simulink model "system_input_18a"  (R2018a)
settings: Solver=FixedStepAuto  StartTime=0.0  StopTime=95  FixedStep=0.05  RelTol=1e-3
libraries: simulink x1
settings Model: Creator=zeiph  LastModifiedBy=zeiph
settings DataIOCC: ReturnWorkspaceOutputs=on
settings SFSimCC: SimUseLocalCustomCode=on
settings RTWCC: RTWUseLocalCustomCode=on

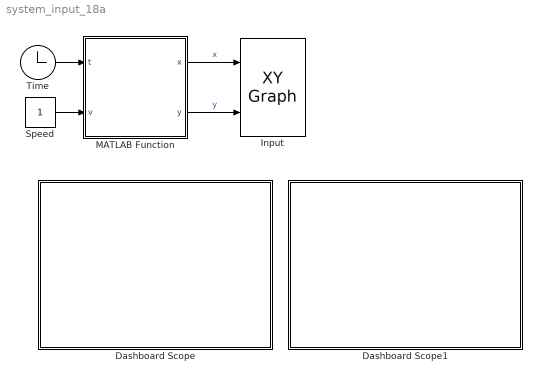
== system system_input_18a ==
  Dashboard Scope : Subsystem  DialogController=hmiCreateDDGDialog  IsWebBlock=on  mask(MWDashboardBlock){webBlockId=c4dcd67c-61d0-45f4-9390-1c8481d4d7a9, webBlockType=sdiscope, ShowInLibBrowser=on, ShowInitialText=on, HMISrcModelName=system_input_18a}
      mask prompts: webBlockId "WebBlock Id"; webBlockType "WebBlock Type"; HMISrcModelName "Source Model"
      mask help: Traces signals on the dashboard scope during simulation.
      mask Help: helpview([docroot '/mapfiles/simulink.map'], 'hmi_scope')
      mask Display:
      | if strcmp(get_param(bdroot(gcb),'BlockDiagramType'),'library')
      |  image([(matlabroot) '/toolbox/simulink/hmi/icons/SDIScope.png'])
      | end
  Dashboard Scope1 : Subsystem  DialogController=hmiCreateDDGDialog  IsWebBlock=on  mask(MWDashboardBlock){webBlockId=b6572997-c2b8-490f-8907-67e1a082daec, webBlockType=sdiscope, ShowInLibBrowser=on, ShowInitialText=on, HMISrcModelName=system_input_18a}
      mask prompts: webBlockId "WebBlock Id"; webBlockType "WebBlock Type"; HMISrcModelName "Source Model"
      mask help: Traces signals on the dashboard scope during simulation.
      mask Help: helpview([docroot '/mapfiles/simulink.map'], 'hmi_scope')
      mask Display:
      | if strcmp(get_param(bdroot(gcb),'BlockDiagramType'),'library')
      |  image([(matlabroot) '/toolbox/simulink/hmi/icons/SDIScope.png'])
      | end
  Input : simulink/Sinks/XY Graph  xmin=-0.1  xmax=5.5  ymin=-5  ymax=13  st=-1
  MATLAB Function : MATLAB Function  TreatAsAtomicUnit=on
  Speed : Constant
  Time : Clock
  wires:
  Time/1 -> MATLAB Function/1(t)
  MATLAB Function/1(x) -> Input/1  "x"
  MATLAB Function/2(y) -> Input/2  "y"
  Speed/1 -> MATLAB Function/2(v)

== system system_input_18a/Dashboard Scope ==

== system system_input_18a/Dashboard Scope1 ==

== matlab function system_input_18a/MATLAB Function ==
  data: x output; t input; y output; v input
function [x , y] = input(t , v)

    h = 10; %Straight line distance
    d = 5; %"Circle" diameter

    
    t = (mod(t , 2*h/v + 2*(d/v))); %% Loop

    is_on_part_1_flag = (t <= h/v);
    is_on_part_2_flag = (t > h/v && t <= h/v + d/v);
    is_on_part_3_flag = (t > h/v + d/v && t <= (2*h/v)+d/v); 
    is_on_part_4_flag = (~is_on_part_1_flag &&...
                         ~is_on_part_2_flag &&...
                         ~is_on_part_3_flag);
    
    timestamp = (is_on_part_1_flag) * t +...
                (is_on_part_2_flag) * (t - h/v) + ... 
                (is_on_part_3_flag) * (t - h/v - d/v)+...
                (is_on_part_4_flag) * (t - (2*h/v + (d/v)));


    y = is_on_part_1_flag * (timestamp*v)+...
        is_on_part_2_flag * (h + (d/2) * sin(pi*timestamp*v/d))+... 
        is_on_part_3_flag * (h-timestamp*v)+...
        is_on_part_4_flag * (-(d/2) * sin(pi*timestamp*v/d));

        
    x = is_on_part_1_flag * (0)+...
        is_on_part_2_flag * (timestamp*v)+... 
        is_on_part_3_flag * (d)+...
        is_on_part_4_flag * ((d - timestamp*v >0)*(d - timestamp*v));

            
            


end
